simulink model "urineanalylsis"  (R2022a)
settings: Solver=VariableStepAuto  StartTime=0.0  StopTime=10.0  RelTol=1e-3
undefined symbols (not defined in the file): sigbuilder_block
libraries: simulink x7
settings Model: Creator=user  LastModifiedBy=user

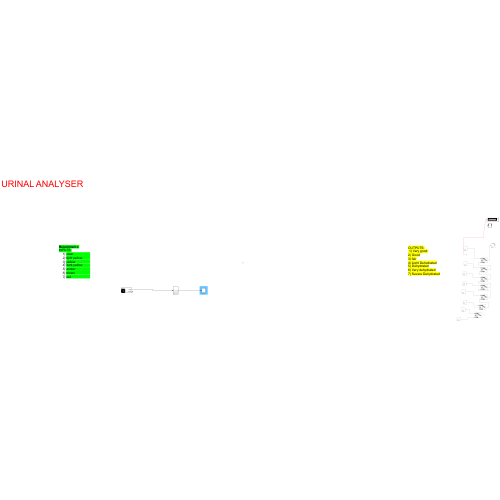
[thumbnail: Simulink's stored preview of the top-level diagram]
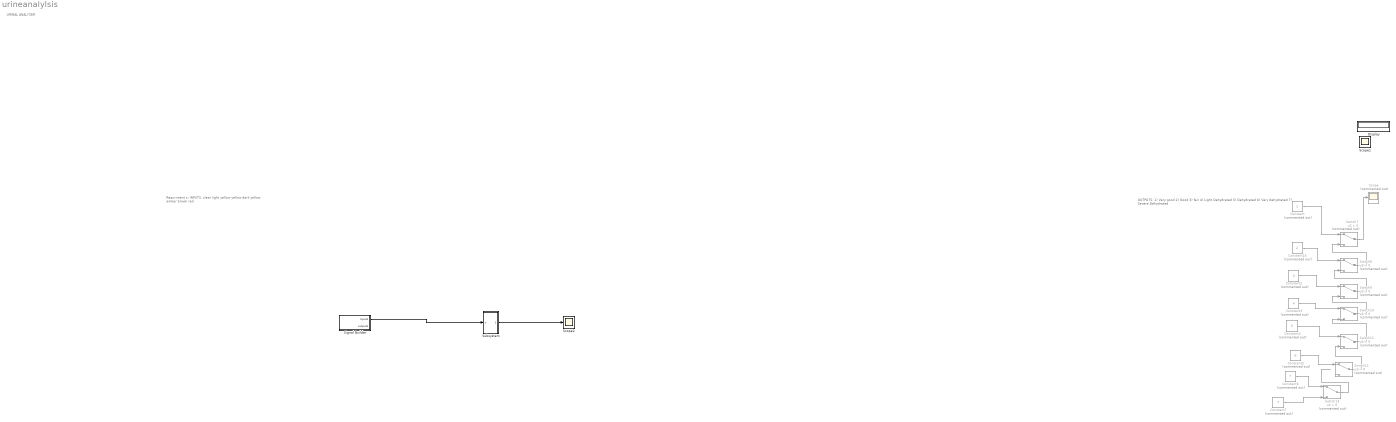
== system urineanalylsis ==
  note: OUTPUTS:
      | 1) Very good
      | 2) Good
      | 3) fair
      | 4) Light Dehydrated
      | 5) Dehydrated
      | 6) Very dehydrated
      | 7) Severe Dehydrated
  note: URINAL ANALYSER
  note: Requriment s:
      | INPUTS:
      | clear
      | light yellow
      | yellow
      | dark yellow
      | amber
      | brown
      | red
  Constant : Constant  Commented=on
  Constant16 : Constant  Commented=on  Value=2
  Constant2 : Constant  Commented=on  Value=3
  Constant3 : Constant  Commented=on  Value=4
  Constant4 : Constant  Commented=on  Value=5
  Constant5 : Constant  Commented=on  Value=6
  Constant6 : Constant  Commented=on  Value=7
  Constant7 : Constant  Commented=on  Value=7
  Display : Display
  Scope : Scope  Commented=on
  Scope1 : Scope
  Scope2 : Scope
  Signal Builder : Subsystem  Tag=STV Subsys  LoadFcn=sigbuilder_block('load');  StartFcn=sigbuilder_block('start');  StopFcn=sigbuilder_block('stop');  ClipboardFcn=sigbuilder_block('clipboard');  mask(Sigbuilder block){tuvar=[0:10]}
      mask help: Simulink:masks:SigbuilderBlock_MD
      mask init:
      | if ~strcmp(get_param(bdroot(gcbh),'SimulationStatus'),'stopped') tuvar = sigbuilder_block('maskInit'); end
      settings: CopyFcn=sigbuilder_block('copy');  DeleteFcn=sigbuilder_block('delete');  ModelCloseFcn=sigbuilder_block('modelClose');  PreSaveFcn=sigbuilder_block('preSave');  PauseFcn=sigbuilder_block('pause');  ContinueFcn=sigbuilder_block('continue');  NameChangeFcn=sigbuilder_block('namechange');  OpenFcn=sigbuilder_block('open',[0 30 1024.5 488.25 ]);  CloseFcn=sigbuilder_block('close');
      mask Display: plot(0, 0, 100, 100,[2, 2, 32, 32, 2], [68, 8, 8, 68, 68],[32, 2], [38, 38], [32, 19, 2],[53, 60, 44], [32, 17, 17, 2],[16, 16, 31, 31]);txt = getActiveGroup(gcbh);text(2, 100, txt,'verticalAlignment', 'top');
  Subsystem : Subsystem
  Switch{7..13} (7 alike) : Switch  Commented=on  Criteria=u2 > Threshold  SaturateOnIntegerOverflow=off  InputSameDT=off
  wires:
  ? -> ?
  ? -> Display/1
  Switch7/1 -> Scope/1
  Constant2/1 -> Switch9/1
  Constant3/1 -> Switch10/1
  Switch12/1 -> Switch11/3
  Switch8/1 -> Switch7/3
  Constant16/1 -> Switch8/1
  Constant4/1 -> Switch11/1
  Switch11/1 -> Switch10/3
  Switch9/1 -> Switch8/3
  Switch13/1 -> ?
  Constant/1 -> Switch7/1
  Constant5/1 -> Switch12/1
  Switch10/1 -> Switch9/3
  Constant6/1 -> Switch13/1
  Constant7/1 -> Switch13/3
  Signal Builder/1(inputs) -> Subsystem/1(u)
  Subsystem/1(Out1) -> Scope2/1

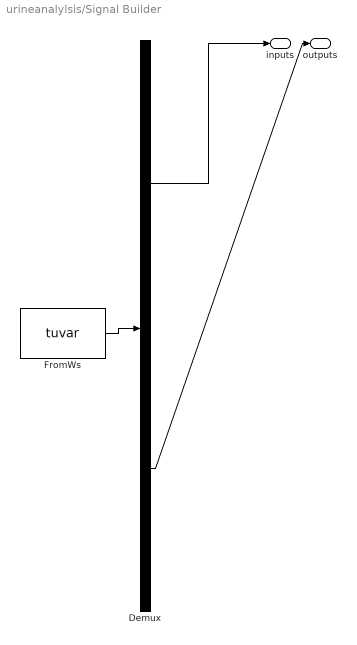
== system urineanalylsis/Signal Builder ==
  Demux : Demux  Tag=STV Demux  Outputs=2
      settings: DisplayOption=none
  FromWs : FromWorkspace  Tag=STV FromWs  VariableName=tuvar
      SigBuilderData=|
      | common.afterFinalStr = 'Extrapolate'
      | common.sampleTime = 0
      | dataSet.timeRange = [1 7]
      | dataSet.name = 'Sheet1'
      | sbobj.Name = 'Signal Builder'
      | sbobj.Groups.Name = 'Sheet1'
      | sbobj.Groups.Signals(1).Name = 'inputs'
      | sbobj.Groups.Signals(1).XData = [1 2 3 4 5 6 7]
      | sbobj.Groups.Signals(1).YData = [1 2 3 4 5 6 7]
      | sbobj.Groups.Signals(2).Name = 'outputs'
      | sbobj.Groups.Signals(2).XData = [1 2 3 4 5 6 7]
      | sbobj.Groups.Signals(2).YData = [1 2 3 4 5 6 7]
      | sbobj.Groups.TimeRange = [1 7]
  inputs : Outport  Tag=STV Outport
  outputs : Outport  Tag=STV Outport  Port=2
  wires:
  Demux/1 -> inputs/1
  FromWs/1 -> Demux/1
  Demux/2 -> outputs/1

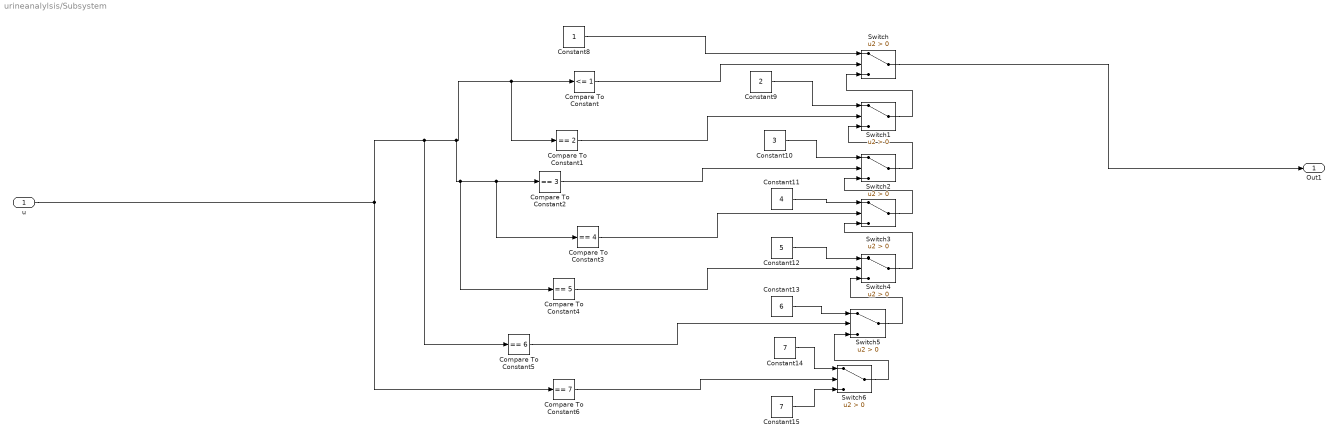
== system urineanalylsis/Subsystem ==
  u : Inport
  Compare To Constant : simulink/Logic and Bit Operations/Compare To Constant  relop=<=  const=1  OutDataTypeStr=boolean
  Compare To Constant1 : simulink/Logic and Bit Operations/Compare To Constant  relop===  const=2  OutDataTypeStr=boolean
  Compare To Constant2 : simulink/Logic and Bit Operations/Compare To Constant  relop===  const=3  OutDataTypeStr=boolean
  Compare To Constant3 : simulink/Logic and Bit Operations/Compare To Constant  relop===  const=4  OutDataTypeStr=boolean
  Compare To Constant4 : simulink/Logic and Bit Operations/Compare To Constant  relop===  const=5  OutDataTypeStr=boolean
  Compare To Constant5 : simulink/Logic and Bit Operations/Compare To Constant  relop===  const=6  OutDataTypeStr=boolean
  Compare To Constant6 : simulink/Logic and Bit Operations/Compare To Constant  relop===  const=7  OutDataTypeStr=boolean
  Constant10 : Constant  Value=3
  Constant11 : Constant  Value=4
  Constant12 : Constant  Value=5
  Constant13 : Constant  Value=6
  Constant14 : Constant  Value=7
  Constant15 : Constant  Value=7
  Constant8 : Constant
  Constant9 : Constant  Value=2
  Switch{,1..6} (7 alike) : Switch  Criteria=u2 > Threshold  SaturateOnIntegerOverflow=off  InputSameDT=off
  Out1 : Outport
  wires:
  u/1 -> Compare To Constant5/1, Compare To Constant4/1, Compare To Constant3/1, Compare To Constant2/1, Compare To Constant1/1, Compare To Constant/1, Compare To Constant6/1
  Constant12/1 -> Switch4/1
  Switch4/1 -> Switch3/3
  Compare To Constant5/1 -> Switch5/2
  Compare To Constant6/1 -> Switch6/2
  Compare To Constant2/1 -> Switch2/2
  Constant14/1 -> Switch6/1
  Compare To Constant/1 -> Switch/2
  Constant9/1 -> Switch1/1
  Constant15/1 -> Switch6/3
  Compare To Constant3/1 -> Switch3/2
  Constant13/1 -> Switch5/1
  Constant10/1 -> Switch2/1
  Constant11/1 -> Switch3/1
  Constant8/1 -> Switch/1
  Switch3/1 -> Switch2/3
  Switch1/1 -> Switch/3
  Switch6/1 -> Switch5/3
  Switch5/1 -> Switch4/3
  Switch2/1 -> Switch1/3
  Compare To Constant4/1 -> Switch4/2
  Compare To Constant1/1 -> Switch1/2
  Switch/1 -> Out1/1
